simulink model "parellel"  (R2020a)
settings: Solver=VariableStepAuto  StartTime=0.0  StopTime=5  RelTol=1e-3
settings Model: EnablePacing=on  PacingRate=0.320000  Creator=I3  LastModifiedBy=I3

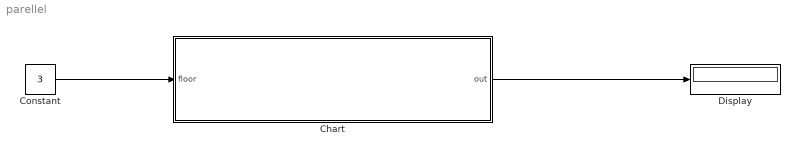
== system parellel ==
  Chart : Stateflow chart  TreatAsAtomicUnit=on
  Constant : Constant  Value=3
  Display : Display
  wires:
  Chart/1(out) -> Display/1
  Constant/1 -> Chart/1(floor)

== stateflow chart parellel/Chart ==
  state active [parallel]
    settings: executionOrder=1
    state stop
      out=current;
    state up
      entry:
      current=0;
      du:
      current=current+1;
    state down
      entry:
      current=0;
      du:
      current=current-1;
    (default) -> stop : {current=1;}
    stop -> stop [order 1] : [floor==current]
    stop -> up [order 2] : [current<floor]
    stop -> down [order 3] : [current>floor]
    up -> stop [order 1] : [current==floor]
    down -> stop : [current==floor]
    up -> up [order 2] : [current<floor]
  state floor [parallel]
    settings: executionOrder=2
    state s2
      entry:
      out=2;
      current=out;
    state s1
      entry:
      current=1;
      out=1;
    state s3
      entry:
      out=3;
      current=out;
    state s4
      entry:
      out=4;
      current=out;
    state s5
      entry:
      out=5;
      current=out;
    s1 -> s1 [order 2] : [current==floor]
    (default) -> s1
    s1 -> s2 [order 1] : [current<floor]
    s4 -> s3 [order 2] : [current>floor]
    s2 -> s3 [order 1] : [current<floor]
    s2 -> s1 [order 2] : [current>floor]
    s3 -> s2 [order 2] : [current>floor]
    s3 -> s4 [order 1] : [current<floor]
    s5 -> s4 [order 1] : [current>floor]
    s4 -> s5 [order 1] : [current<floor]
    s5 -> s5 [order 2] : [floor==current]
  data: floor input; out output; current local
